simulink model "Motor_Step_Response"  (R2020b)
settings: Solver=VariableStepAuto  StartTime=0.0  StopTime=10.0  RelTol=1e-9
undefined symbols (not defined in the file): Jm, KcRa, Km, N_n, V_step, x0
libraries: simulink x1
settings Model: Creator=domin  LastModifiedBy=domin

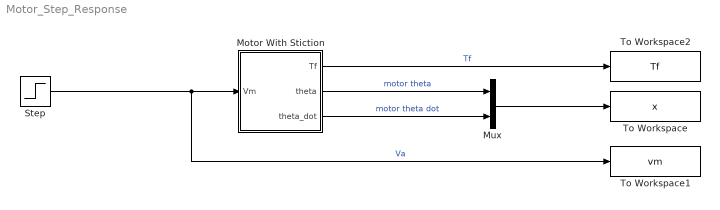
== system Motor_Step_Response ==
  " Motor With Stiction" : Subsystem
  Mux : Mux  Inputs=2
  Step : Step  Time=0  After=V_step  SampleTime=0
  To Workspace : ToWorkspace  VariableName=x  SampleTime=-1
  To Workspace1 : ToWorkspace  VariableName=vm  SampleTime=-1
  To Workspace2 : ToWorkspace  VariableName=Tf  SampleTime=-1
  wires:
  " Motor With Stiction"/1(Tf) -> To Workspace2/1  "Tf"
  " Motor With Stiction"/2(theta) -> Mux/1  "motor theta"
  Mux/1 -> To Workspace/1
  " Motor With Stiction"/3(theta_dot) -> Mux/2  "motor theta dot"
  Step/1 -> To Workspace1/1, " Motor With Stiction"/1(Vm)  "Va"

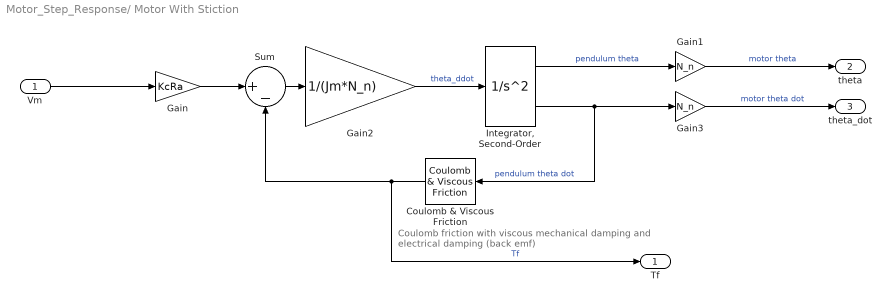
== system Motor_Step_Response/ Motor With Stiction ==
  note: Coulomb friction with viscous mechanical damping
      | and electrical damping (back emf)
  Vm : Inport
  Coulomb & Viscous Friction : simulink/Discontinuities/Coulomb & Viscous Friction  offset=T_ba  gain=N_n*KcRa/Km
  Gain : Gain  Gain=KcRa
  Gain1 : Gain  Gain=N_n
  Gain2 : Gain  Gain=1/(Jm*N_n)
  Gain3 : Gain  Gain=N_n
  "Integrator, Second-Order" : SecondOrderIntegrator  ICX=x0(1)  ICDXDT=x0(2)  ZeroCross=off
  Sum : Sum  Inputs=|+-
  Tf : Outport
  theta : Outport  Port=2
  theta_dot : Outport  Port=3
  wires:
  Gain2/1 -> "Integrator, Second-Order"/1  "theta_ddot"
  "Integrator, Second-Order"/2 -> Gain3/1, Coulomb & Viscous Friction/1  "pendulum theta dot"
  Coulomb & Viscous Friction/1 -> Sum/2, Tf/1  "Tf"
  "Integrator, Second-Order"/1 -> Gain1/1  "pendulum theta"
  Sum/1 -> Gain2/1
  Vm/1 -> Gain/1
  Gain/1 -> Sum/1
  Gain1/1 -> theta/1  "motor theta"
  Gain3/1 -> theta_dot/1  "motor theta dot"
